simulink model "sixDOF"  (R2026a)
settings: Solver=ode4  StopTime=30  FixedStep=0.001
values from neighbouring files (symbols this model uses):
  Cd = [1.038104 1.038104 1.038104 1.038104 1.038104 1.038104 1.038104 1.038113 0.680861 0.53385 0.46574 0.427146 ... (523 elements, 523x1)]    [dragcurve.mat]
  cg_or = [1.246677 1.246275 1.245672 1.244766 1.243402 1.241498 1.239584 1.23766 1.236081 1.234015 1.231937 1.229847 ... (503 elements, 503x1)]    [rocketMassProps.mat]
  cp_or = [1.422105 1.424498 1.427709 1.432664 1.438361 1.443278 1.448387 1.4529 1.45482 1.458116 1.462888 1.467443 ... (503 elements, 503x1)]    [rocketMassProps.mat]
  CP_shift_table = [0 0.02 0.05 0.09 0.14]    [Cpvsdep.m]    (also in cpShiftData.mat)
  deployPct_table = [0 25 50 75 100]    [Cpvsdep.m]    (also in cpShiftData.mat)
  Ixx_or = [0.041252 0.041245 0.041234 0.041218 0.041194 0.04116 0.041126 0.041092 0.041064 0.041028 0.040992 0.040956 ... (503 elements, 503x1)]    [rocketMassProps.mat]
  Iyy_or = [7.47729 7.471945 7.463917 7.45185 7.433695 7.408377 7.382931 7.357357 7.336389 7.308965 7.281391 7.253668 ... (503 elements, 503x1)]    [rocketMassProps.mat]
  mass_or = [17.606951 17.596657 17.581217 17.558056 17.523315 17.475074 17.426833 17.378591 17.33922 17.287969 17.236717 17.185466 ... (503 elements, 503x1)]    [rocketMassProps.mat]
  thrust = [0 100 1500 2000 2200 1800 1950 2034 2000 1900 1760 1700 ... (16 elements, 16x1)]    [thrustcurve.mat]
  time = [0 0.055 0.092 0.1 0.15 0.2 0.5 1 1.5 2 2.5 2.9 ... (16 elements, 16x1)]    [thrustcurve.mat]
  time_c = [0 0.01 0.02 0.03 0.04 0.05 0.055 0.0625 0.0725 0.0825 0.092 0.1 ... (523 elements, 523x1)]    [dragcurve.mat]
  time_or = [0.222509 0.233178 0.249181 0.273186 0.309194 0.359194 0.409194 0.459194 0.5 0.55 0.6 0.65 ... (503 elements, 503x1)]    [rocketMassProps.mat]
libraries: simulink x4, sharedTrackingLibrary x1
settings Model: LastModifiedBy=Lenovo

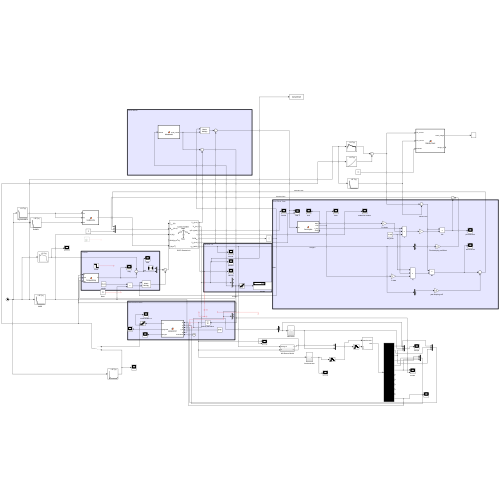
[thumbnail: Simulink's stored preview of the top-level diagram]
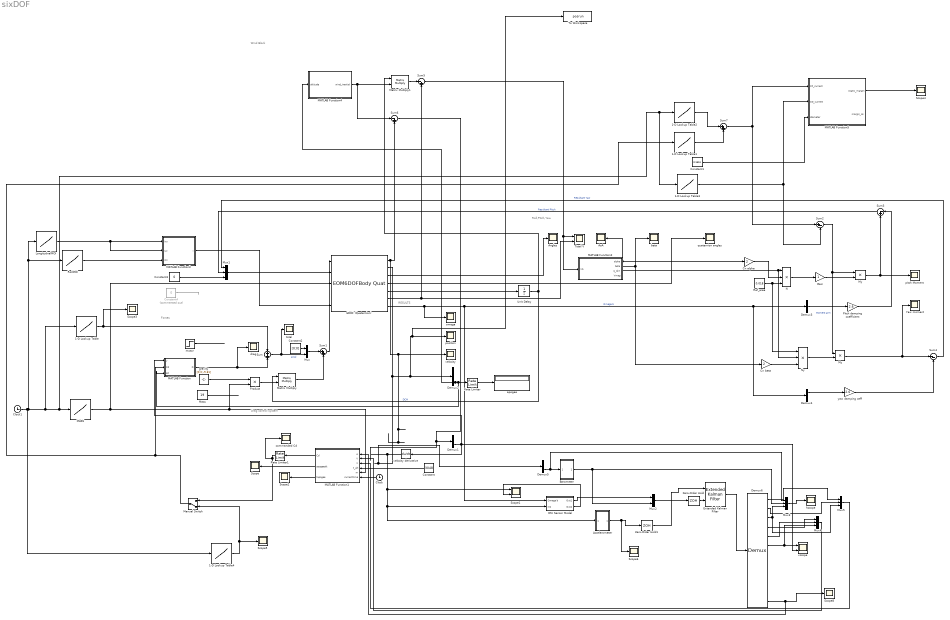
== system sixDOF ==
  note: Wind Block
  note: RESULTS
  note: Roll,Pitch,Yaw
  note: Drag control system
  note: Forces
  1-D Lookup Table : Lookup_n-D  NumberOfTableDimensions=1  BreakpointsForDimension1=time  Table=thrust  ExtrapMethod=Clip  UseLastTableValue=on  InternalRulePriority=Speed  RndMeth=Simplest
  1-D Lookup Table1 : Lookup_n-D  NumberOfTableDimensions=1  BreakpointsForDimension1=deployPct_table  Table=CP_shift_table  InternalRulePriority=Speed  RndMeth=Simplest
  1-D Lookup Table2 : Lookup_n-D  NumberOfTableDimensions=1  BreakpointsForDimension1=time_or  Table=cp_or  ExtrapMethod=Clip  InternalRulePriority=Speed  RndMeth=Simplest
  1-D Lookup Table3 : Lookup_n-D  NumberOfTableDimensions=1  BreakpointsForDimension1=time_or  Table=cg_or  ExtrapMethod=Clip  InternalRulePriority=Speed  RndMeth=Simplest
  1-D Lookup Table4 : Lookup_n-D  NumberOfTableDimensions=1  BreakpointsForDimension1=time_c  Table=Cd  ExtrapMethod=Clip  InternalRulePriority=Speed  RndMeth=Simplest
  6DOF (Quaternion) : EOM6DOFBodyQuat  mtype=Custom Variable  mass_0=19
  Accelerometer : Subsystem
  Angles : Scope
      settings: ActiveDisplayYMinimum=-0.38622595750085542  ActiveDisplayYMaximum=1.7735495845731737  DataLoggingVariableName=ScopeData8
  AoA : Scope
      settings: ActiveDisplayYMinimum=-0.11670515236456694  ActiveDisplayYMaximum=0.1972270518440222  DataLoggingVariableName=ScopeData7
  Barometer : Subsystem
  Clock : Clock
  Clock1 : Clock
  Cn alpha : Gain  Gain=2
  Cn beta : Gain  Gain=2
  Constant : Constant  Value=3048
  Constant1 : Constant  Value=0.1524
  Constant2 : Constant  Value=[0;0]
  Constant3 : Constant  Value=0
  Constant4 : Constant  Commented=on  Value=0
  Demux{1..5} (5 alike) : Demux  Outputs=3
  Demux6 : Demux  Outputs=12
  Extended Kalman Filter : sharedTrackingLibrary/Extended Kalman Filter  StateTransitionFcn=StateTransitionFcn  HasStateTransitionJacobianFcn=off  HasAdditiveProcessNoise=Additive  ProcessNoise=Q_matrix  HasTimeVaryingProcessNoise=off  HasStateTransitionFcnExtraArgument=1  InitialState=zeros(12,1)  InitialStateCovariance=eye(12)*0.1  MeasurementFcn1=MeasurementFcn  HasMeasurementJacobianFcn1=off  HasMeasurementEnablePort1=off  HasAdditiveMeasurementNoise1=Additive  MeasurementNoise1=R_matrix  HasTimeVaryingMeasurementNoise1=off  HasMeasurementFcnExtraArgument1=0  HasMeasurementWrapping1=off  HasMeasurementJacobianFcn2=off  HasMeasurementEnablePort2=off  HasAdditiveMeasurementNoise2=Additive  MeasurementNoise2=1  HasTimeVaryingMeasurementNoise2=off  HasMeasurementFcnExtraArgument2=0  HasMeasurementWrapping2=off  HasMeasurementJacobianFcn3=off  HasMeasurementEnablePort3=off  HasAdditiveMeasurementNoise3=Additive  MeasurementNoise3=1  HasTimeVaryingMeasurementNoise3=off  HasMeasurementFcnExtraArgument3=0  HasMeasurementWrapping3=off  HasMeasurementJacobianFcn4=off  HasMeasurementEnablePort4=off  HasAdditiveMeasurementNoise4=Additive  MeasurementNoise4=1  HasTimeVaryingMeasurementNoise4=off  HasMeasurementFcnExtraArgument4=0  HasMeasurementWrapping4=off  HasMeasurementJacobianFcn5=off  HasMeasurementEnablePort5=off  HasAdditiveMeasurementNoise5=Additive  MeasurementNoise5=1  HasTimeVaryingMeasurementNoise5=off  HasMeasurementFcnExtraArgument5=0  HasMeasurementWrapping5=off  EnableMultirate=off  StateTransitionFcnSampleTime=1  MeasurementFcn1SampleTime=1  MeasurementFcn2SampleTime=1  MeasurementFcn3SampleTime=1  MeasurementFcn4SampleTime=1  MeasurementFcn5SampleTime=1  UseCurrentEstimator=on  OutputStateCovariance=off  DataType=double  SampleTime=0.001  NumberOfMeasurements=1
  Gain : Gain
  IMU Sensor Model : Subsystem
  LongitudnalMOI : Lookup_n-D  NumberOfTableDimensions=1  BreakpointsForDimension1=time_or  Table=Iyy_or  ExtrapMethod=Clip  InternalRulePriority=Speed  RndMeth=Simplest
  MASS : Lookup_n-D  NumberOfTableDimensions=1  BreakpointsForDimension1=time_or  Table=mass_or  ExtrapMethod=Clip  InternalRulePriority=Speed  RndMeth=Simplest
  MATLAB Function : MATLAB Function  TreatAsAtomicUnit=on
  MATLAB Function1 : MATLAB Function  TreatAsAtomicUnit=on
  MATLAB Function2 : MATLAB Function  TreatAsAtomicUnit=on
  MATLAB Function3 : MATLAB Function  TreatAsAtomicUnit=on
  MATLAB Function4 : MATLAB Function  TreatAsAtomicUnit=on
  MATLAB Function5 : MATLAB Function  TreatAsAtomicUnit=on
  Manual Switch : ManualSwitch  CurrentSetting=0
  Mass : Constant  Value=19
  Matrix Multiply : Product  Multiplication=Matrix(*)
  Matrix Multiply1 : Product  Multiplication=Matrix(*)
  Mux : Mux  Inputs=2
  Mux{1,3..5} (4 alike) : Mux  Inputs=3
  Mux2 : Mux  Inputs=2
  My : Product
  Mz : Product
  N : Product  Inputs=3
  Ny : Product  Inputs=3
  Pitch damping coefficient : Gain  Gain=2.6
  Product : Product
  Rate Limiter : RateLimiter  RisingSlewLimit=99999  FallingSlewLimit=0  SampleTimeMode=inherited
  Rate Limiter1 : RateLimiter  RisingSlewLimit=0.8  FallingSlewLimit=-0.8  SampleTimeMode=inherited
  Ref_area : Constant  Value=0.018
  RollMOI : Lookup_n-D  NumberOfTableDimensions=1  BreakpointsForDimension1=time_or  Table=Ixx_or  ExtrapMethod=Clip  InternalRulePriority=Speed  RndMeth=Simplest
  Scope{,2..6,8} (7 alike) : Scope
      Scope settings: ActiveDisplayYMinimum=-3975.2759341657311  ActiveDisplayYMaximum=5346.1757277784072  DataLoggingVariableName=ScopeData4
      Scope2 settings: ActiveDisplayYMinimum=23.131664202979607  ActiveDisplayYMaximum=34.456731548921958  DataLoggingVariableName=ScopeData6
      Scope3 settings: ActiveDisplayYMinimum=-765.07484589225214  ActiveDisplayYMaximum=2519.6031220028276  DataLoggingVariableName=ScopeData15
      Scope4 settings: ActiveDisplayYMinimum=1.5294476200072862  ActiveDisplayYMaximum=1.5909519727413044  DataLoggingVariableName=ScopeData20
      Scope5 settings: DataLoggingVariableName=ScopeData21
      Scope6 settings: ActiveDisplayYMinimum=-108.72602500762326  ActiveDisplayYMaximum=165.70364248889467  DataLoggingVariableName=ScopeData22
      Scope8 settings: ActiveDisplayYMinimum=-91.088508044335612  ActiveDisplayYMaximum=61.000475305282336  DataLoggingVariableName=ScopeData23
  Scope1 : Scope  NumInputPorts=2
      settings: ActiveDisplayYMinimum=-195.213202209058  ActiveDisplayYMaximum=201.78596327672926  DataLoggingVariableName=ScopeData16
  Sum : Sum
  Sum1 : Sum  Inputs=|++
  Sum2 : Sum  Inputs=|+-
  Sum3 : Sum  Inputs=|-+
  Sum4 : Sum  Inputs=|--
  Sum5 : Sum  Inputs=|-+
  Sum6 : Sum  Inputs=|-+
  Sum7 : Sum  Inputs=|++
  To Workspace : ToWorkspace  VariableName=posrun  SampleTime=-1
  Total V : Scope  NumInputPorts=2
      settings: ActiveDisplayYMinimum=-119.83899710725643  ActiveDisplayYMaximum=265.49667563260067  DataLoggingVariableName=ScopeData11
  Unit Delay : UnitDelay  SampleTime=-1
  Yaw moment : Scope
      settings: ActiveDisplayYMinimum=-18.650703940874124  ActiveDisplayYMaximum=20.0541694649058  DataLoggingVariableName=ScopeData12
  Zero-Order Hold : ZeroOrderHold  SampleTime=0.001
  Zero-Order Hold1 : ZeroOrderHold  SampleTime=0.001
  apogee : Display
  beta : Scope
      settings: ActiveDisplayYMinimum=-0.79579174295748067  ActiveDisplayYMaximum=0.81085505135714131  DataLoggingVariableName=ScopeData13
  commanded Cd : Scope
      settings: ActiveDisplayYMinimum=0.34716611962376021  ActiveDisplayYMaximum=1.5460260105933847  DataLoggingVariableName=ScopeData5
  drag : Scope
      settings: ActiveDisplayYMinimum=-396.86130675218692  ActiveDisplayYMaximum=62.412916979427223  DataLoggingVariableName=ScopeData2
  gravity : Constant  Value=[0;0;-9.81]  VectorParams1D=off
  hscope : Scope
      settings: ActiveDisplayYMinimum=3031.207782140717  ActiveDisplayYMaximum=3036.9094424347427  DataLoggingVariableName=ScopeData17
  motor : Step  Time=3.6  InitialValue=1667.8  FinalValue=0  SampleTime=0
  omega : Scope
      settings: ActiveDisplayYMinimum=-1.5223393973231611  ActiveDisplayYMaximum=1.5244987566500803  DataLoggingVariableName=ScopeData9
  pitch Moment : Scope
      settings: ActiveDisplayYMinimum=-72.212026662162884  ActiveDisplayYMaximum=251.70727276885549  DataLoggingVariableName=ScopeData10
  position : Scope
      settings: ActiveDisplayYMinimum=0.81729052010257419  ActiveDisplayYMaximum=1635.7826927369022
  quaternion angles : Scope
      settings: ActiveDisplayYMinimum=-1.2402927428054364  ActiveDisplayYMaximum=1.2489214158672706  DataLoggingVariableName=ScopeData14
  total : Scope
      settings: ActiveDisplayYMinimum=-148.90644792235315  ActiveDisplayYMaximum=814.83016826926712  DataLoggingVariableName=ScopeData3
  velocity : Scope
      settings: ActiveDisplayYMinimum=-83.67558276135  ActiveDisplayYMaximum=165.81112772987149
  velocity derivative : Derivative
  vscope : Scope  NumInputPorts=2
      settings: ActiveDisplayYMinimum=156.86344831807537  ActiveDisplayYMaximum=238.92304472262  DataLoggingVariableName=ScopeData18
  yaw damping ceff : Gain  Gain=2.6
  wires:
  motor/1 -> ?
  MATLAB Function/1(D) -> Sum/2, drag/1
  Sum/1 -> Mux/2, total/1  "axial"
  6DOF (Quaternion)/1 -> velocity/1, Sum6/2
  Demux1/3 -> vscope/2, MATLAB Function/1(v), velocity derivative/1
  velocity derivative/1 -> Scope1/1, Accelerometer/1(In1), IMU Sensor Model/2(In2)
  Constant/1 -> MATLAB Function1/4(t_alt)
  Clock/1 -> MATLAB Function1/6(currenttime)
  MATLAB Function1/1(Cd) -> Rate Limiter1/1
  Rate Limiter/1 -> apogee/1
  Demux2/3 -> MATLAB Function/3(alt), Rate Limiter/1, MATLAB Function4/1(altitude)
  Manual Switch/1 -> 1-D Lookup Table1/1, MATLAB Function/2(Cd)
  MATLAB Function1/2(apogeealt) -> Scope/1
  MATLAB Function1/3(tapogee) -> Scope2/1
  Sum1/1 -> 6DOF (Quaternion)/1
  gravity/1 -> Product/1
  Mass/1 -> ?
  Product/1 -> Matrix Multiply/2
  6DOF (Quaternion)/5 -> Unit Delay/1
  Unit Delay/1 -> Matrix Multiply1/1, Matrix Multiply/1  "DCM"
  Matrix Multiply/1 -> Sum1/2
  Constant2/1 -> Mux/1
  Mux/1 -> Sum1/1
  Mux1/1 -> 6DOF (Quaternion)/2
  6DOF (Quaternion)/6 -> Total V/2, Sum5/2
  MATLAB Function2/1(alpha) -> Cn alpha/1, AoA/1
  MATLAB Function2/3(q_dyn) -> Ny/2, N/1
  Cn alpha/1 -> N/2
  Ref_area/1 -> N/3, Ny/1
  Sum7/1 -> Sum2/1, MATLAB Function5/1(CP_current)
  1-D Lookup Table3/1 -> Sum2/2, MATLAB Function5/2(CG_current)
  Sum2/1 -> My/1, Mz/1  "Moment arm"
  N/1 -> Gain/1
  Constant4/1 -> ?
  My/1 -> Sum3/2, pitch Moment/1
  6DOF (Quaternion)/3 -> Angles/1
  6DOF (Quaternion)/7 -> Demux3/1, Demux4/1, IMU Sensor Model/1(Omega b), omega/1  "Omega b"
  Gain/1 -> My/2
  Demux3/2 -> Pitch damping coefficient/1
  Pitch damping coefficient/1 -> Sum3/1
  Sum3/1 -> Mux1/2  "Resultant Pitch"
  Ny/1 -> Mz/2
  Mz/1 -> Sum4/1, Yaw moment/1
  MATLAB Function2/2(beta) -> beta/1, Cn beta/1
  Cn beta/1 -> Ny/3
  Constant3/1 -> Mux1/3
  Demux4/1 -> yaw damping ceff/1
  Sum4/1 -> Mux1/1  "Resultant Yaw"
  6DOF (Quaternion)/4 -> quaternion angles/1
  yaw damping ceff/1 -> Sum4/2
  MASS/1 -> Product/2, MATLAB Function1/5(m), 6DOF (Quaternion)/3
  LongitudnalMOI/1 -> MATLAB Function3/2(Iyy), MATLAB Function3/1(Ixx)
  RollMOI/1 -> MATLAB Function3/3(Izz)
  MATLAB Function3/1(I) -> 6DOF (Quaternion)/5
  1-D Lookup Table/1 -> Scope3/1, Sum/1
  IMU Sensor Model/2(Out2) -> Scope1/2
  Demux5/3 -> Mux3/1, Barometer/1(In1)
  Barometer/1(Out1) -> Mux2/2, Mux3/2
  Mux2/1 -> Zero-Order Hold/1
  Zero-Order Hold/1 -> Extended Kalman Filter/2
  Extended Kalman Filter/1 -> Demux6/1
  Demux6/3 -> Mux5/3, Mux3/3
  Mux3/1 -> hscope/1
  IMU Sensor Model/1(Out1) -> Mux2/1
  Accelerometer/1(Out1) -> Scope6/1, Zero-Order Hold1/1
  Zero-Order Hold1/1 -> Extended Kalman Filter/1
  MATLAB Function4/1(wind_inertial) -> Sum6/1, Matrix Multiply1/2
  Matrix Multiply1/1 -> Sum5/1
  Sum5/1 -> Total V/1, MATLAB Function2/1(Vb)
  Sum6/1 -> Demux1/1
  Demux6/6 -> Mux4/3, vscope/1
  1-D Lookup Table2/1 -> Sum7/1
  1-D Lookup Table1/1 -> Sum7/2
  Constant1/1 -> MATLAB Function5/3(diameter)
  MATLAB Function5/1(static_margin) -> Scope4/1
  6DOF (Quaternion)/2 -> Demux5/1, To Workspace/1, position/1, Demux2/1
  1-D Lookup Table4/1 -> Scope5/1, Manual Switch/2
  Rate Limiter1/1 -> commanded Cd/1, Manual Switch/1
  Clock1/1 -> 1-D Lookup Table4/1, 1-D Lookup Table3/1, 1-D Lookup Table2/1, MASS/1, 1-D Lookup Table/1, RollMOI/1, LongitudnalMOI/1
  Demux6/12 -> MATLAB Function1/1(A), Scope8/1
  ? -> ?
  Demux6/4 -> Mux4/1
  Demux6/5 -> Mux4/2
  Mux4/1 -> MATLAB Function1/2(V)
  Demux6/1 -> Mux5/1
  Demux6/2 -> Mux5/2
  Mux5/1 -> MATLAB Function1/3(X)

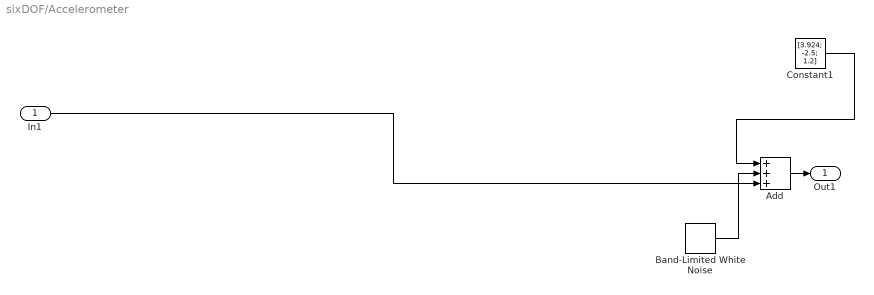
== system sixDOF/Accelerometer ==
  In1 : Inport
  Add : Sum  Inputs=+++
  Band-Limited White Noise : simulink/Sources/Band-Limited White Noise  Cov=[0.00012; 0.00012; 0.00012]  Ts=0.001  seed=[23341]
  Constant1 : Constant  Value=[3.924; -2.5; 1.2]
  Out1 : Outport
  wires:
  Band-Limited White Noise/1 -> Add/2
  Add/1 -> Out1/1
  Constant1/1 -> Add/1
  In1/1 -> Add/3

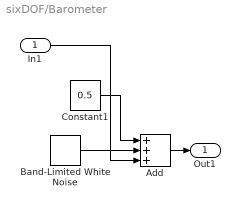
== system sixDOF/Barometer ==
  In1 : Inport
  Add : Sum  Inputs=+++
  Band-Limited White Noise : simulink/Sources/Band-Limited White Noise  Cov=[0.00001]  Ts=0.001  seed=[23341]
  Constant1 : Constant  Value=0.5
  Out1 : Outport
  wires:
  Band-Limited White Noise/1 -> Add/2
  Constant1/1 -> Add/1
  Add/1 -> Out1/1
  In1/1 -> Add/3

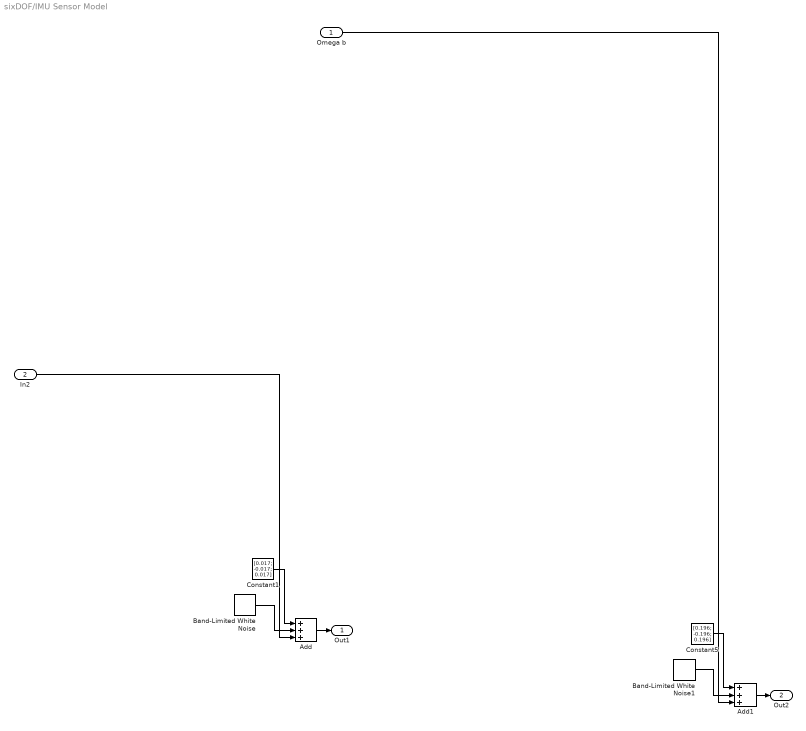
== system sixDOF/IMU Sensor Model ==
  Omega b : Inport
  In2 : Inport  Port=2
  Add : Sum  Inputs=+++
  Add1 : Sum  Inputs=+++
  Band-Limited White Noise : simulink/Sources/Band-Limited White Noise  Cov=[0.0000000000048; 0.0000000000048; 0.0000000000048]  Ts=0.001  seed=[23341]
  Band-Limited White Noise1 : simulink/Sources/Band-Limited White Noise  Cov=[0.00000000047; 0.00000000047; 0.00000000047]  Ts=0.001  seed=[23341]
  Constant1 : Constant  Value=[0.017; -0.017; 0.017]
  Constant5 : Constant  Value=[0.196; -0.196; 0.196]
  Out1 : Outport
  Out2 : Outport  Port=2
  wires:
  In2/1 -> Add/3
  Constant5/1 -> Add1/1
  Band-Limited White Noise/1 -> Add/2
  Band-Limited White Noise1/1 -> Add1/2
  Add1/1 -> Out2/1
  Constant1/1 -> Add/1
  Omega b/1 -> Add1/3
  Add/1 -> Out1/1

== matlab function sixDOF/MATLAB Function1 ==
  data: Cd output; apogeealt output; tapogee output; A input; V input; X input; t_alt input; m input; currenttime input
function [Cd,apogeealt,tapogee] = apogeepred(A,V,X,t_alt,m,currenttime)

apogeeTG = t_alt;

currentAlt= X(3);

currentverticalvel=V(3);

currentverticalacc=A;

persistent alt_lut rho_lut

if isempty(alt_lut)

S = coder.load('atmoData.mat');

alt_lut = S.altitude_data;

rho_lut = S.density_data;

end

Area = 0.018;

Cdclean = 0.3;

vsim = currentverticalvel;

altsim = currentAlt;

t = currenttime;

deltat = 0.01;

apogeealt = 0;

tapogee=0;

if(currentverticalacc > 0)

Cd=Cdclean;

return;

end

    
for c = 1:10

Cdsim= Cdclean + c*0.08;

for i = 1 : 3000

rho = interp1(alt_lut, rho_lut, altsim, 'linear', 'extrap');

F = -0.5*Cdsim*rho*Area*(vsim^2) - 9.81*m;

asim= F/m;

vsim = vsim + asim*deltat;

altsim = altsim + vsim*deltat;

t=t+deltat;

if(vsim<0)

apogeealt=altsim;

tapogee = t;

break;

end

end

Cd=Cdsim;

if apogeealt < apogeeTG

break;

end

end

== matlab function sixDOF/MATLAB Function ==
  data: v input; D output; Cd input; alt input
function D = ComputeDrag(v,Cd,alt)
A=0.018;
altsim = alt;
persistent alt_lut rho_lut
if isempty(alt_lut)

    S = coder.load('atmoData.mat');

    alt_lut = S.altitude_data;

    rho_lut = S.density_data;

end
rho = interp1(alt_lut, rho_lut, altsim, 'linear', 'extrap');
%Cd=0.3;

D = -0.5*Cd*rho*A*(v^2);
end

== matlab function sixDOF/MATLAB Function2 ==
  data: Vb input; alpha output; beta output; q_dyn output; Vmag output
function [alpha,beta, q_dyn, Vmag] = AeroAngles(Vb)
    u = Vb(1); v = Vb(2); w = Vb(3);
    Vmag = sqrt(u^2 + v^2 + w^2);
    
    if Vmag < 0.1
        alpha = 0;
        beta = 0;
    else
        alpha = atan2(u, w);
        beta = atan2(v,w);
    end
    
    rho = 1.225;   
    q_dyn = 0.5*rho*Vmag^2;
end

== matlab function sixDOF/MATLAB Function3 ==
  data: Ixx input; I output; Iyy input; Izz input
function I = buildInertia(Ixx, Iyy, Izz)
    I = diag([Ixx, Iyy, Izz]);
end

== matlab function sixDOF/MATLAB Function4 ==
  data: altitude input; wind_inertial output
function wind_inertial = WindModel(altitude)
    v_ref = 5;      
    h_ref = 10;     
    alpha_shear = 0.14;   

    if altitude < 1
        alt_calc = 1;  
    else
        alt_calc = altitude;
    end

    wind_speed = v_ref * (alt_calc/h_ref)^alpha_shear;

    wind_inertial = [wind_speed; 0; 0];
end

== matlab function sixDOF/MATLAB Function5 ==
  data: CP_current input; static_margin output; CG_current input; diameter input; margin_ok output
function [static_margin, margin_ok] = StabilityCheck(CP_current, CG_current, diameter)
    static_margin = (CP_current - CG_current) / diameter;
    margin_ok = (static_margin >= 1.5) && (static_margin <= 2.5);
end
